simulink model "sim_mpc_lmi"  (Simulink 8.2)
settings: Solver=ode4  SolverMode=SingleTasking  StartTime=0.0  StopTime=10  FixedStep=0.01  RelTol=1e-3
values from neighbouring files (symbols this model uses):
  A = [0 1;-2 -3]    [ex1.m]
  Ac = [0 1;0 0]    [ex2.m]
  Bc = [0;1]    [ex2.m]
  C = [1 0]    [ex2.m]
  T = 1    [ex2.m]
undefined symbols (not defined in the file or in its folder): B
settings Model: Creator=Kawakami  LastModifiedBy=Eduardo
settings DataIOCC: LimitDataPoints=off  SaveOutput=off  SaveTime=off  TimeSaveName=t  SignalLoggingName=sigsOut
settings OptimizationCC: BooleanDataType=off
settings DebuggingCC: SaveWithParameterizedLinksMsg=none  SignalResolutionControl=TryResolveAllWithWarning  SolverPrmCheckMsg=none  MultiTaskDSMMsg=warning  MultiTaskCondExecSysMsg=none
settings HardwareCC: TargetUnknown=on
settings RTWCC: IncludeERTFirstTime=on

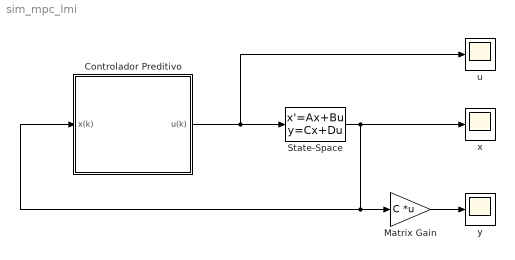
== system sim_mpc_lmi ==
  "Controlador Preditivo  " : Subsystem  mask{A=A, B=B, C=C, S=[1 0;0 1], R=1, umax=1*1000, ymax=0.5*1000, T=T}
  Matrix Gain : Gain  Gain=C  Multiplication=Matrix(K*u)  SaturateOnIntegerOverflow=on  OutDataTypeStr=Inherit: Same as input  ParamDataTypeStr=Inherit: Same as input
  State-Space : StateSpace  A=Ac  B=Bc  C=eye(size(Ac,1))  D=zeros(size(Ac,1),size(Bc,2))  X0=[2;1]
  u : Scope
      settings: TimeRange=10  YMin=-2  YMax=0.5
  x : Scope
      settings: YMin=-1.25  YMax=2.25
  y : Scope
      settings: TimeRange=10  YMin=-1  YMax=1  SaveName=ScopeData2
  wires:
  "Controlador Preditivo  "/1(u(k)) -> State-Space/1, u/1
  State-Space/1 -> x/1, "Controlador Preditivo  "/1(x(k)), Matrix Gain/1
  Matrix Gain/1 -> y/1

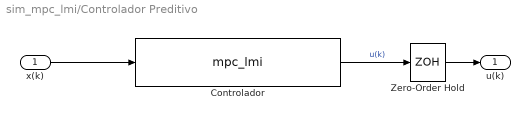
== system sim_mpc_lmi/Controlador Preditivo   ==
  x(k) : Inport
  Controlador : S-Function  FunctionName=mpc_lmi  Parameters=S,R,A,B,C,umax,ymax,T  EnableBusSupport=off
  Zero-Order Hold : ZeroOrderHold  SampleTime=T
  u(k) : Outport
  wires:
  Zero-Order Hold/1 -> u(k)/1
  Controlador/1 -> Zero-Order Hold/1  "u(k)"
  x(k)/1 -> Controlador/1
